simulink model "D2C_01_Asservissement_Position"  (R2018b)
settings: Solver=ode45  StartTime=0.0  StopTime=20  FixedStep=0.003  RelTol=1e-3  EnableMultiTasking=on
libraries: slctrlblks x2, simulink x1
settings Model: Creator=Propriétaire  LastModifiedBy=xpess
settings DataIOCC: LimitDataPoints=on  SaveFormat=Array  SignalLoggingSaveFormat=ModelDataLogs
settings OptimizationCC: ExpressionDepthLimit=2147483647  LifeSpan=inf
settings DebuggingCC: UnderspecifiedInitializationDetection=Classic  MergeDetectMultiDrivingBlocksExec=none  SolverPrmCheckMsg=warning  FcnCallInpInsideContextMsg=warning  StateNameClashWarn=warning  SFUnexpectedBacktrackingDiag=warning  SFNoUnconditionalDefaultTransitionDiag=warning  SFExecutionAtInitializationDiag=none
settings HardwareCC: ProdBitPerPointer=32  ProdBitPerSizeT=32  ProdBitPerPtrDiffT=32  ProdLargestAtomicFloat=None  ProdIntDivRoundTo=Undefined  ProdEndianess=Unspecified  ProdWordSize=32  ProdHWDeviceType=32-bit Generic
settings ModelReferenceCC: PropagateSignalLabelsOutOfModel=off
settings SFSimCC: SimUseLocalCustomCode=off
settings RTWCC: RTWUseLocalCustomCode=off
settings CodeAppCC: StateflowObjectComments=on
settings GRTTargetCC: TargetLangStandard=C89/C90 (ANSI)  GeneratePreprocessorConditionals=Disable all  CombineOutputUpdateFcns=off  GRTInterface=on
settings ConfigComp: CovMetricSettings=dw  CovHtmlReporting=on  CovSaveCumulativeToWorkspaceVar=on  CovSaveSingleToWorkspaceVar=on  CovExternalEMLEnable=off

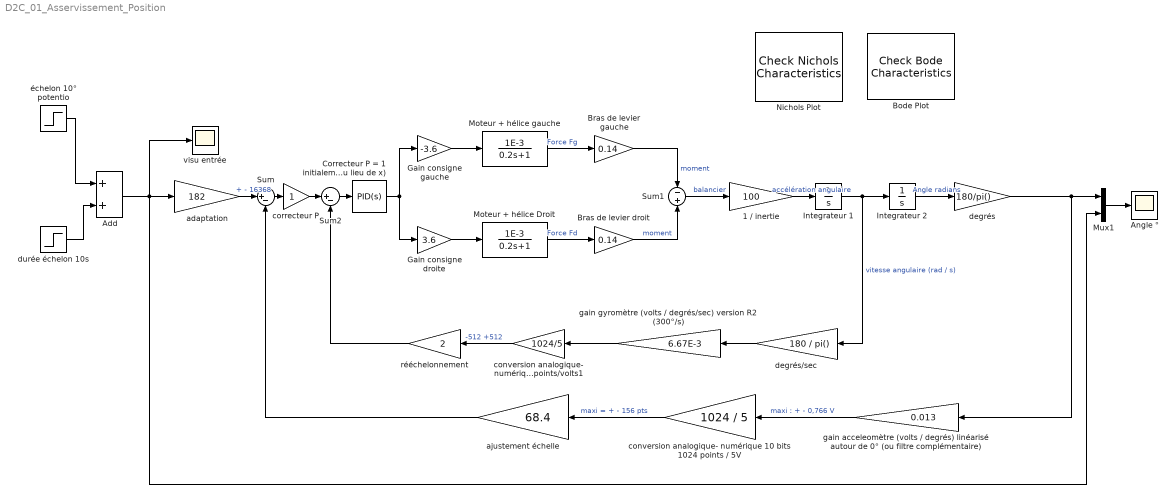
== system D2C_01_Asservissement_Position ==
  1 / inertie : Gain  Gain=100
  Add : Sum
  Angle ° : Scope
  Bode Plot : slctrlblks/Model Verification/Check Bode  Characteristics  InstantiateOnLoad=on  SaveOperatingPoints=off  LinearizationIOs={'/Sum', 1, 'in', 'on', '';'/ajustement échelle', 1, 'out', 'on', ''}  LinearizeAt=SnapshotTimes  SnapshotTimes=[0]  TriggerType=rising  SampleTime=auto  RateConversionMethod=zoh  PreWarpFreq=10  UseExactDelayModel=off  UseFullBlockNameLabels=off  UseBusSignalLabels=off  enabled=on  stopWhenAssertionFail=off  export=off  ViewDlgPos=[100 200 510 390]  OpenViewOnLoad=off  LaunchViewOnOpen=on  FrequencyUnits=rad/s  MagnitudeUnits=dB  PhaseUnits=deg  TimeUnits=seconds  EnableUpperBound=off  UpperBoundFrequencies=[]  UpperBoundMagnitudes=[]  EnableLowerBound=off  LowerBoundFrequencies=[]  LowerBoundMagnitudes=[]
      settings: SourceProductName=Simulink Control Design
  Bras de levier droit : Gain  Gain=0.14
  Bras de levier gauche : Gain  Gain=0.14
  "Correcteur P = 1 initialement (attention pour Kd : utiliser x/50 au lieu de x)" : simulink/Continuous/PID Controller  Controller=PID  Form=Parallel  TimeDomain=Continuous-time  SampleTime=1  IntegratorMethod=Forward Euler  FilterMethod=Forward Euler  ControllerParametersSource=internal  P=1  I=0  D=0  UseFilter=on  N=50  TunerSelectOption=Transfer Function Based (PID Tuner App)  InitialConditionSource=internal  InitialConditionForIntegrator=0  InitialConditionForFilter=0  DifferentiatorICPrevScaledInput=0  ExternalReset=none  TrackingMode=off  Kt=1  LimitOutput=off  UpperSaturationLimit=inf  LowerSaturationLimit=-inf  LinearizeAsGain=on  AntiWindupMode=none  Kb=1  POutMin=[]  POutMax=[]  IOutMin=[]  IOutMax=[]  DOutMin=[]  DOutMax=[]  NOutMin=[]  NOutMax=[]  SumOutMin=[]  SumOutMax=[]  SaturationOutMin=[]  SaturationOutMax=[]  PParamMin=[]  PParamMax=[]  IParamMin=[]  IParamMax=[]  DParamMin=[]  DParamMax=[]  NParamMin=[]  NParamMax=[]  KbParamMin=[]  KbParamMax=[]  KtParamMin=[]  KtParamMax=[]  KbOutMin=[]  KbOutMax=[]  KtOutMin=[]  KtOutMax=[]  IntegratorOutMin=[]  IntegratorOutMax=[]  FilterOutMin=[]  FilterOutMax=[]  SumI1OutMin=[]  SumI1OutMax=[]  SumI2OutMin=[]  SumI2OutMax=[]  SumI3OutMin=[]  SumI3OutMax=[]  SumI4OutMin=[]  SumI4OutMax=[]  SumDOutMin=[]  SumDOutMax=[]  DifferentiatorOutMin=[]  DifferentiatorOutMax=[]  FilterDiffOutCoefMin=[]  FilterDiffOutCoefMax=[]  ReciprocalOutMin=[]  ReciprocalOutMax=[]  SumDenOutMin=[]  SumDenOutMax=[]  SumNumOutMin=[]  SumNumOutMax=[]  DivideOutMin=[]  DivideOutMax=[]  IntegratorContinuousStateAttributes=''  IntegratorStateMustResolveToSignalObject=off  IntegratorRTWStateStorageClass=Auto  FilterContinuousStateAttributes=''  FilterStateMustResolveToSignalObject=off  FilterRTWStateStorageClass=Auto  ParallelPVariant=InternalParameters  IdealPVariant=Disabled  IVariant=InternalParameters  DVariant=InternalParameters  IntegratorVariant=Continuous  SatVariant=Disabled  AWVariant=Passthrough  PCopyVariant=Disabled  TRVariant=Disabled  FdbkBlocksVariant=Forward  IdealPFdbkVariant=Disabled  SatFdbkVariant=Disabled  DerivativeFilterVariant=ContFilter  NVariant=InternalParameters  NCopyVariant=Disabled  FilterICVariant=InternalICsFilter  IntegratorICVariant=InternalICs  ExternalResetVariant=Disabled  TRSumVariant=Passthrough  SumFdbkVariant=Disabled  SumVariant=Sum_PID
  Gain consigne droite : Gain  Gain=3.6
  Gain consigne gauche : Gain  Gain=-3.6
  Integrateur 1 : Integrator
  Integrateur 2 : Integrator
  Moteur + hélice Droit : TransferFcn  Numerator=[1E-3]  Denominator=[0.2 1]
  Moteur + hélice gauche : TransferFcn  Numerator=[1E-3]  Denominator=[0.2 1]
  Mux1 : Mux  Inputs=2
  Nichols Plot : slctrlblks/Model Verification/Check Nichols Characteristics  InstantiateOnLoad=on  SaveOperatingPoints=off  LinearizationIOs={'/Sum', 1, 'in', 'on', '';'/ajustement échelle', 1, 'out', 'on', ''}  LinearizeAt=SnapshotTimes  SnapshotTimes=[0]  TriggerType=rising  SampleTime=auto  RateConversionMethod=zoh  PreWarpFreq=10  UseExactDelayModel=off  UseFullBlockNameLabels=off  UseBusSignalLabels=off  enabled=on  stopWhenAssertionFail=off  export=off  ViewDlgPos=[100 200 510 390]  LaunchViewOnOpen=on  OpenViewOnLoad=off  FrequencyUnits=rad/s  MagnitudeUnits=dB  PhaseUnits=deg  TimeUnits=seconds  EnableMargins=off  GainMargin=[]  PhaseMargin=[]  EnableGainPhaseBound=off  GainPhaseBoundType={'upper'}  OLPhases=[]  OLGains=[]  EnableCLPeakGain=off  CLPeakGain=[]  FeedbackSign=-1
      settings: SourceProductName=Simulink Control Design  SourceProductBaseCode=SD  SaveToWorkspace=off  SaveName=sys
  Sum : Sum  Inputs=|+-
  Sum1 : Sum  Inputs=-|+
  Sum2 : Sum  Inputs=|+-
  adaptation : Gain  Gain=182
  ajustement échelle : Gain  Gain=68.4
  conversion analogique- numérique points/volts1 : Gain  Gain=1024/5
  conversion analogique- numérique 10 bits 1024 points / 5V : Gain  Gain=1024 / 5
  correcteur P : Gain
  degrés : Gain  Gain=180/pi()
  degrés/sec : Gain  Gain=180 / pi()
  durée échelon 10s : Step  Time=10  After=-10  SampleTime=0
  gain acceleomètre (volts / degrés) linéarisé autour de 0° (ou filtre complémentaire) : Gain  Gain=0.013
  gain gyromètre (volts / degrés/sec) version R2 (300°/s) : Gain  Gain=6.67E-3
  rééchelonnement : Gain  Gain=2
  visu entrée : Scope
  échelon 10° potentio : Step  Time=0  After=10  SampleTime=0
  wires:
  Moteur + hélice gauche/1 -> Bras de levier gauche/1  "Force Fg"
  Bras de levier gauche/1 -> Sum1/1  "moment"
  Moteur + hélice Droit/1 -> Bras de levier droit/1  "Force Fd"
  Bras de levier droit/1 -> Sum1/2  "moment"
  Gain consigne gauche/1 -> Moteur + hélice gauche/1
  Gain consigne droite/1 -> Moteur + hélice Droit/1
  Sum1/1 -> 1 / inertie/1  "balancier"
  gain acceleomètre (volts / degrés) linéarisé autour de 0° (ou filtre complémentaire)/1 -> conversion analogique- numérique 10 bits 1024 points / 5V/1  "maxi : + - 0,766 V"
  Integrateur 2/1 -> degrés/1  "Angle radians"
  1 / inertie/1 -> Integrateur 1/1  "accélération angulaire"
  adaptation/1 -> Sum/1  "+ - 16368"
  degrés/1 -> gain acceleomètre (volts / degrés) linéarisé autour de 0° (ou filtre complémentaire)/1, Mux1/1
  Add/1 -> visu entrée/1, Mux1/2, adaptation/1
  échelon 10° potentio/1 -> Add/1
  durée échelon 10s/1 -> Add/2
  conversion analogique- numérique 10 bits 1024 points / 5V/1 -> ajustement échelle/1  "maxi = + - 156 pts"
  Mux1/1 -> Angle °/1
  ajustement échelle/1 -> Sum/2
  Sum/1 -> correcteur P/1
  Integrateur 1/1 -> degrés/sec/1, Integrateur 2/1  "vitesse angulaire (rad / s)"
  conversion analogique- numérique points/volts1/1 -> rééchelonnement/1  "-512 +512"
  degrés/sec/1 -> gain gyromètre (volts / degrés/sec) version R2 (300°/s)/1
  gain gyromètre (volts / degrés/sec) version R2 (300°/s)/1 -> conversion analogique- numérique points/volts1/1
  "Correcteur P = 1 initialement (attention pour Kd : utiliser x/50 au lieu de x)"/1 -> Gain consigne droite/1, Gain consigne gauche/1
  correcteur P/1 -> Sum2/1
  Sum2/1 -> "Correcteur P = 1 initialement (attention pour Kd : utiliser x/50 au lieu de x)"/1
  rééchelonnement/1 -> Sum2/2
